simulink model "UR5_CB3_admittance_template"  (R2020b)
settings: Solver=FixedStepAuto  StartTime=0.0  StopTime=30  FixedStep=1/500  MaxStep=1e-2  RelTol=1e-3
model workspace: external: MATLAB File UR5_CB3Params.m (data not in the file)
values from neighbouring files (symbols this model uses):
  a = [0 -0.425 -0.39225 0 0 0]    [UR5_CB3Params.m]
  alpha = [1.5707963267948966 0 0 1.5707963267948966 -1.5707963267948966           0]    [UR5_CB3Params.m]
  d = [0.089159 0 0 0.10915 0.09465 0.0823]    [UR5_CB3Params.m]
  m1 = 3.7    [UR5_CB3Params.m]
  m2 = 8.393    [UR5_CB3Params.m]
  m3 = 2.33    [UR5_CB3Params.m]
  m4 = 1.219    [UR5_CB3Params.m]
  m5 = 1.219    [UR5_CB3Params.m]
  m6 = 0.1879    [UR5_CB3Params.m]
  q0 = [1;1;1;1;1;1]    [UR5_CB3Params.m]
  UR5_CB3Data = struct    [UR5_CB3Params.m]
undefined symbols (not defined in the file or in its folder): Do, Kd, Ko, Kp, Md, Mo, X, Y, Z
libraries: sm_lib x154, nesl_utility x19
(part 3 of 3)

== system UR5_CB3_admittance_template/UR5 (CB3)/Link 3/Link 3/x31101_Support_14_RIGID ==
  ReferenceFrame : sm_lib/Frames and Transforms/Reference Frame
  Solid : sm_lib/Body Elements/File Solid  ExtGeomFileName=31101_Support_ipt_da604d82.STEP  UnitType=FromFile  ExtGeomFileUnits=m  StepReaderType=HEX  ExportConvexHullGeometry=off  InertiaType=Custom  Mass=UR5_CB3Data.Solid(8).mass  MassUnits=lbm  CenterOfMass=UR5_CB3Data.Solid(8).CoM  CenterOfMassUnits=mm  MomentsOfInertia=UR5_CB3Data.Solid(8).MoI  MomentsOfInertiaUnits=lbm*mm^2  ProductsOfInertia=UR5_CB3Data.Solid(8).PoI  ProductsOfInertiaUnits=lbm*mm^2  BasedOnType=Density  Density=1000  DensityUnits=kg/m^3  DoExposeReferenceFrame=on  SerializedFrames=<Frames/>  GraphicType=FromGeometry  MarkerShape=Sphere  MarkerSize=10  GraphicVisPropType=SimpleVisualProperties  GraphicDiffuseColor=UR5_CB3Data.Solid(8).color  GraphicSpecularColor=[0.5 0.5 0.5 1.0]  GraphicAmbientColor=[0.15 0.15 0.15 1.0]  GraphicEmissiveColor=[0.0 0.0 0.0 1.0]  GraphicShininess=75  GraphicOpacity=UR5_CB3Data.Solid(8).opacity
  F : PMIOPort  Side=Left
  connections:
  Solid/RConn1 -- ReferenceFrame/RConn1 -- F/RConn1

== system UR5_CB3_admittance_template/UR5 (CB3)/Link 3/Link 3/x31105_Support_24_RIGID ==
  ReferenceFrame : sm_lib/Frames and Transforms/Reference Frame
  Solid : sm_lib/Body Elements/File Solid  ExtGeomFileName=31105_Support_ipt_79716e66.STEP  UnitType=FromFile  ExtGeomFileUnits=m  StepReaderType=HEX  ExportConvexHullGeometry=off  InertiaType=Custom  Mass=UR5_CB3Data.Solid(12).mass  MassUnits=lbm  CenterOfMass=UR5_CB3Data.Solid(12).CoM  CenterOfMassUnits=mm  MomentsOfInertia=UR5_CB3Data.Solid(12).MoI  MomentsOfInertiaUnits=lbm*mm^2  ProductsOfInertia=UR5_CB3Data.Solid(12).PoI  ProductsOfInertiaUnits=lbm*mm^2  BasedOnType=Density  Density=1000  DensityUnits=kg/m^3  DoExposeReferenceFrame=on  SerializedFrames=<Frames/>  GraphicType=FromGeometry  MarkerShape=Sphere  MarkerSize=10  GraphicVisPropType=SimpleVisualProperties  GraphicDiffuseColor=UR5_CB3Data.Solid(12).color  GraphicSpecularColor=[0.5 0.5 0.5 1.0]  GraphicAmbientColor=[0.15 0.15 0.15 1.0]  GraphicEmissiveColor=[0.0 0.0 0.0 1.0]  GraphicShininess=75  GraphicOpacity=UR5_CB3Data.Solid(12).opacity
  F : PMIOPort  Side=Left
  connections:
  Solid/RConn1 -- ReferenceFrame/RConn1 -- F/RConn1

== system UR5_CB3_admittance_template/UR5 (CB3)/Link 3/Link 3/x31106_Support_13_RIGID ==
  ReferenceFrame : sm_lib/Frames and Transforms/Reference Frame
  Solid : sm_lib/Body Elements/File Solid  ExtGeomFileName=31106_Support_ipt_3245b488.STEP  UnitType=FromFile  ExtGeomFileUnits=m  StepReaderType=HEX  ExportConvexHullGeometry=off  InertiaType=Custom  Mass=UR5_CB3Data.Solid(7).mass  MassUnits=lbm  CenterOfMass=UR5_CB3Data.Solid(7).CoM  CenterOfMassUnits=mm  MomentsOfInertia=UR5_CB3Data.Solid(7).MoI  MomentsOfInertiaUnits=lbm*mm^2  ProductsOfInertia=UR5_CB3Data.Solid(7).PoI  ProductsOfInertiaUnits=lbm*mm^2  BasedOnType=Density  Density=1000  DensityUnits=kg/m^3  DoExposeReferenceFrame=on  SerializedFrames=<Frames/>  GraphicType=FromGeometry  MarkerShape=Sphere  MarkerSize=10  GraphicVisPropType=SimpleVisualProperties  GraphicDiffuseColor=UR5_CB3Data.Solid(7).color  GraphicSpecularColor=[0.5 0.5 0.5 1.0]  GraphicAmbientColor=[0.15 0.15 0.15 1.0]  GraphicEmissiveColor=[0.0 0.0 0.0 1.0]  GraphicShininess=75  GraphicOpacity=UR5_CB3Data.Solid(7).opacity
  F : PMIOPort  Side=Left
  connections:
  Solid/RConn1 -- ReferenceFrame/RConn1 -- F/RConn1

== system UR5_CB3_admittance_template/UR5 (CB3)/Link 3/Link 3/x31362_Support_27_RIGID ==
  ReferenceFrame : sm_lib/Frames and Transforms/Reference Frame
  Solid : sm_lib/Body Elements/File Solid  ExtGeomFileName=31362_Support_ipt_dfed11ef.STEP  UnitType=FromFile  ExtGeomFileUnits=m  StepReaderType=HEX  ExportConvexHullGeometry=off  InertiaType=Custom  Mass=UR5_CB3Data.Solid(14).mass  MassUnits=lbm  CenterOfMass=UR5_CB3Data.Solid(14).CoM  CenterOfMassUnits=mm  MomentsOfInertia=UR5_CB3Data.Solid(14).MoI  MomentsOfInertiaUnits=lbm*mm^2  ProductsOfInertia=UR5_CB3Data.Solid(14).PoI  ProductsOfInertiaUnits=lbm*mm^2  BasedOnType=Density  Density=1000  DensityUnits=kg/m^3  DoExposeReferenceFrame=on  SerializedFrames=<Frames/>  GraphicType=FromGeometry  MarkerShape=Sphere  MarkerSize=10  GraphicVisPropType=SimpleVisualProperties  GraphicDiffuseColor=UR5_CB3Data.Solid(14).color  GraphicSpecularColor=[0.5 0.5 0.5 1.0]  GraphicAmbientColor=[0.15 0.15 0.15 1.0]  GraphicEmissiveColor=[0.0 0.0 0.0 1.0]  GraphicShininess=75  GraphicOpacity=UR5_CB3Data.Solid(14).opacity
  F : PMIOPort  Side=Left
  connections:
  Solid/RConn1 -- ReferenceFrame/RConn1 -- F/RConn1

== system UR5_CB3_admittance_template/UR5 (CB3)/Link 3/Link 3/x33115_Support_32_RIGID ==
  ReferenceFrame : sm_lib/Frames and Transforms/Reference Frame
  Solid : sm_lib/Body Elements/File Solid  ExtGeomFileName=33115_Support_ipt_5ce5d1d.STEP  UnitType=FromFile  ExtGeomFileUnits=m  StepReaderType=HEX  ExportConvexHullGeometry=off  InertiaType=Custom  Mass=UR5_CB3Data.Solid(16).mass  MassUnits=lbm  CenterOfMass=UR5_CB3Data.Solid(16).CoM  CenterOfMassUnits=mm  MomentsOfInertia=UR5_CB3Data.Solid(16).MoI  MomentsOfInertiaUnits=lbm*mm^2  ProductsOfInertia=UR5_CB3Data.Solid(16).PoI  ProductsOfInertiaUnits=lbm*mm^2  BasedOnType=Density  Density=1000  DensityUnits=kg/m^3  DoExposeReferenceFrame=on  SerializedFrames=<Frames/>  GraphicType=FromGeometry  MarkerShape=Sphere  MarkerSize=10  GraphicVisPropType=SimpleVisualProperties  GraphicDiffuseColor=UR5_CB3Data.Solid(16).color  GraphicSpecularColor=[0.5 0.5 0.5 1.0]  GraphicAmbientColor=[0.15 0.15 0.15 1.0]  GraphicEmissiveColor=[0.0 0.0 0.0 1.0]  GraphicShininess=75  GraphicOpacity=UR5_CB3Data.Solid(16).opacity
  F : PMIOPort  Side=Left
  connections:
  Solid/RConn1 -- ReferenceFrame/RConn1 -- F/RConn1

== system UR5_CB3_admittance_template/UR5 (CB3)/Link 3/Link 3/x33116_Support_31_RIGID ==
  ReferenceFrame : sm_lib/Frames and Transforms/Reference Frame
  Solid : sm_lib/Body Elements/File Solid  ExtGeomFileName=33116_Support_ipt_643963fc.STEP  UnitType=FromFile  ExtGeomFileUnits=m  StepReaderType=HEX  ExportConvexHullGeometry=off  InertiaType=Custom  Mass=UR5_CB3Data.Solid(15).mass  MassUnits=lbm  CenterOfMass=UR5_CB3Data.Solid(15).CoM  CenterOfMassUnits=mm  MomentsOfInertia=UR5_CB3Data.Solid(15).MoI  MomentsOfInertiaUnits=lbm*mm^2  ProductsOfInertia=UR5_CB3Data.Solid(15).PoI  ProductsOfInertiaUnits=lbm*mm^2  BasedOnType=Density  Density=1000  DensityUnits=kg/m^3  DoExposeReferenceFrame=on  SerializedFrames=<Frames/>  GraphicType=FromGeometry  MarkerShape=Sphere  MarkerSize=10  GraphicVisPropType=SimpleVisualProperties  GraphicDiffuseColor=UR5_CB3Data.Solid(15).color  GraphicSpecularColor=[0.5 0.5 0.5 1.0]  GraphicAmbientColor=[0.15 0.15 0.15 1.0]  GraphicEmissiveColor=[0.0 0.0 0.0 1.0]  GraphicShininess=75  GraphicOpacity=UR5_CB3Data.Solid(15).opacity
  F : PMIOPort  Side=Left
  connections:
  Solid/RConn1 -- ReferenceFrame/RConn1 -- F/RConn1

== system UR5_CB3_admittance_template/UR5 (CB3)/Link 3/Link 3/x33303_Support_11_RIGID ==
  ReferenceFrame : sm_lib/Frames and Transforms/Reference Frame
  Solid : sm_lib/Body Elements/File Solid  ExtGeomFileName=33303_Support_ipt_9d9e7990.STEP  UnitType=FromFile  ExtGeomFileUnits=m  StepReaderType=HEX  ExportConvexHullGeometry=off  InertiaType=Custom  Mass=UR5_CB3Data.Solid(2).mass  MassUnits=lbm  CenterOfMass=UR5_CB3Data.Solid(2).CoM  CenterOfMassUnits=mm  MomentsOfInertia=UR5_CB3Data.Solid(2).MoI  MomentsOfInertiaUnits=lbm*mm^2  ProductsOfInertia=UR5_CB3Data.Solid(2).PoI  ProductsOfInertiaUnits=lbm*mm^2  BasedOnType=Density  Density=1000  DensityUnits=kg/m^3  DoExposeReferenceFrame=on  SerializedFrames=<Frames/>  GraphicType=FromGeometry  MarkerShape=Sphere  MarkerSize=10  GraphicVisPropType=SimpleVisualProperties  GraphicDiffuseColor=UR5_CB3Data.Solid(2).color  GraphicSpecularColor=[0.5 0.5 0.5 1.0]  GraphicAmbientColor=[0.15 0.15 0.15 1.0]  GraphicEmissiveColor=[0.0 0.0 0.0 1.0]  GraphicShininess=75  GraphicOpacity=UR5_CB3Data.Solid(2).opacity
  F : PMIOPort  Side=Left
  connections:
  Solid/RConn1 -- ReferenceFrame/RConn1 -- F/RConn1

== system UR5_CB3_admittance_template/UR5 (CB3)/Link 3/Link 3/x34111_Support_15_RIGID ==
  ReferenceFrame : sm_lib/Frames and Transforms/Reference Frame
  Solid : sm_lib/Body Elements/File Solid  ExtGeomFileName=34111_Support_ipt_45739413.STEP  UnitType=FromFile  ExtGeomFileUnits=m  StepReaderType=HEX  ExportConvexHullGeometry=off  InertiaType=Custom  Mass=UR5_CB3Data.Solid(9).mass  MassUnits=lbm  CenterOfMass=UR5_CB3Data.Solid(9).CoM  CenterOfMassUnits=mm  MomentsOfInertia=UR5_CB3Data.Solid(9).MoI  MomentsOfInertiaUnits=lbm*mm^2  ProductsOfInertia=UR5_CB3Data.Solid(9).PoI  ProductsOfInertiaUnits=lbm*mm^2  BasedOnType=Density  Density=1000  DensityUnits=kg/m^3  DoExposeReferenceFrame=on  SerializedFrames=<Frames/>  GraphicType=FromGeometry  MarkerShape=Sphere  MarkerSize=10  GraphicVisPropType=SimpleVisualProperties  GraphicDiffuseColor=UR5_CB3Data.Solid(9).color  GraphicSpecularColor=[0.5 0.5 0.5 1.0]  GraphicAmbientColor=[0.15 0.15 0.15 1.0]  GraphicEmissiveColor=[0.0 0.0 0.0 1.0]  GraphicShininess=75  GraphicOpacity=UR5_CB3Data.Solid(9).opacity
  F : PMIOPort  Side=Left
  connections:
  Solid/RConn1 -- ReferenceFrame/RConn1 -- F/RConn1

== system UR5_CB3_admittance_template/UR5 (CB3)/Link 4/Link 4/x31101_Support_16_RIGID ==
  ReferenceFrame : sm_lib/Frames and Transforms/Reference Frame
  Solid : sm_lib/Body Elements/File Solid  ExtGeomFileName=31101_Support_ipt_da604d82.STEP  UnitType=FromFile  ExtGeomFileUnits=m  StepReaderType=HEX  ExportConvexHullGeometry=off  InertiaType=Custom  Mass=UR5_CB3Data.Solid(8).mass  MassUnits=lbm  CenterOfMass=UR5_CB3Data.Solid(8).CoM  CenterOfMassUnits=mm  MomentsOfInertia=UR5_CB3Data.Solid(8).MoI  MomentsOfInertiaUnits=lbm*mm^2  ProductsOfInertia=UR5_CB3Data.Solid(8).PoI  ProductsOfInertiaUnits=lbm*mm^2  BasedOnType=Density  Density=1000  DensityUnits=kg/m^3  DoExposeReferenceFrame=on  SerializedFrames=<Frames/>  GraphicType=FromGeometry  MarkerShape=Sphere  MarkerSize=10  GraphicVisPropType=SimpleVisualProperties  GraphicDiffuseColor=UR5_CB3Data.Solid(8).color  GraphicSpecularColor=[0.5 0.5 0.5 1.0]  GraphicAmbientColor=[0.15 0.15 0.15 1.0]  GraphicEmissiveColor=[0.0 0.0 0.0 1.0]  GraphicShininess=75  GraphicOpacity=UR5_CB3Data.Solid(8).opacity
  F : PMIOPort  Side=Left
  connections:
  Solid/RConn1 -- ReferenceFrame/RConn1 -- F/RConn1

== system UR5_CB3_admittance_template/UR5 (CB3)/Link 4/Link 4/x31132_Support_25_RIGID ==
  ReferenceFrame : sm_lib/Frames and Transforms/Reference Frame
  Solid : sm_lib/Body Elements/File Solid  ExtGeomFileName=31132_Support_ipt_77457c2f.STEP  UnitType=FromFile  ExtGeomFileUnits=m  StepReaderType=HEX  ExportConvexHullGeometry=off  InertiaType=Custom  Mass=UR5_CB3Data.Solid(13).mass  MassUnits=lbm  CenterOfMass=UR5_CB3Data.Solid(13).CoM  CenterOfMassUnits=mm  MomentsOfInertia=UR5_CB3Data.Solid(13).MoI  MomentsOfInertiaUnits=lbm*mm^2  ProductsOfInertia=UR5_CB3Data.Solid(13).PoI  ProductsOfInertiaUnits=lbm*mm^2  BasedOnType=Density  Density=1000  DensityUnits=kg/m^3  DoExposeReferenceFrame=on  SerializedFrames=<Frames/>  GraphicType=FromGeometry  MarkerShape=Sphere  MarkerSize=10  GraphicVisPropType=SimpleVisualProperties  GraphicDiffuseColor=UR5_CB3Data.Solid(13).color  GraphicSpecularColor=[0.5 0.5 0.5 1.0]  GraphicAmbientColor=[0.15 0.15 0.15 1.0]  GraphicEmissiveColor=[0.0 0.0 0.0 1.0]  GraphicShininess=75  GraphicOpacity=UR5_CB3Data.Solid(13).opacity
  F : PMIOPort  Side=Left
  connections:
  Solid/RConn1 -- ReferenceFrame/RConn1 -- F/RConn1

== system UR5_CB3_admittance_template/UR5 (CB3)/Link 4/Link 4/x33103_Support_20_RIGID ==
  ReferenceFrame : sm_lib/Frames and Transforms/Reference Frame
  Solid : sm_lib/Body Elements/File Solid  ExtGeomFileName=33103_Support_ipt_c3be2011.STEP  UnitType=FromFile  ExtGeomFileUnits=m  StepReaderType=HEX  ExportConvexHullGeometry=off  InertiaType=Custom  Mass=UR5_CB3Data.Solid(10).mass  MassUnits=lbm  CenterOfMass=UR5_CB3Data.Solid(10).CoM  CenterOfMassUnits=mm  MomentsOfInertia=UR5_CB3Data.Solid(10).MoI  MomentsOfInertiaUnits=lbm*mm^2  ProductsOfInertia=UR5_CB3Data.Solid(10).PoI  ProductsOfInertiaUnits=lbm*mm^2  BasedOnType=Density  Density=1000  DensityUnits=kg/m^3  DoExposeReferenceFrame=on  SerializedFrames=<Frames/>  GraphicType=FromGeometry  MarkerShape=Sphere  MarkerSize=10  GraphicVisPropType=SimpleVisualProperties  GraphicDiffuseColor=UR5_CB3Data.Solid(10).color  GraphicSpecularColor=[0.5 0.5 0.5 1.0]  GraphicAmbientColor=[0.15 0.15 0.15 1.0]  GraphicEmissiveColor=[0.0 0.0 0.0 1.0]  GraphicShininess=75  GraphicOpacity=UR5_CB3Data.Solid(10).opacity
  F : PMIOPort  Side=Left
  connections:
  Solid/RConn1 -- ReferenceFrame/RConn1 -- F/RConn1

== system UR5_CB3_admittance_template/UR5 (CB3)/Link 4/Link 4/x33116_Support_30_RIGID ==
  ReferenceFrame : sm_lib/Frames and Transforms/Reference Frame
  Solid : sm_lib/Body Elements/File Solid  ExtGeomFileName=33116_Support_ipt_643963fc.STEP  UnitType=FromFile  ExtGeomFileUnits=m  StepReaderType=HEX  ExportConvexHullGeometry=off  InertiaType=Custom  Mass=UR5_CB3Data.Solid(15).mass  MassUnits=lbm  CenterOfMass=UR5_CB3Data.Solid(15).CoM  CenterOfMassUnits=mm  MomentsOfInertia=UR5_CB3Data.Solid(15).MoI  MomentsOfInertiaUnits=lbm*mm^2  ProductsOfInertia=UR5_CB3Data.Solid(15).PoI  ProductsOfInertiaUnits=lbm*mm^2  BasedOnType=Density  Density=1000  DensityUnits=kg/m^3  DoExposeReferenceFrame=on  SerializedFrames=<Frames/>  GraphicType=FromGeometry  MarkerShape=Sphere  MarkerSize=10  GraphicVisPropType=SimpleVisualProperties  GraphicDiffuseColor=UR5_CB3Data.Solid(15).color  GraphicSpecularColor=[0.5 0.5 0.5 1.0]  GraphicAmbientColor=[0.15 0.15 0.15 1.0]  GraphicEmissiveColor=[0.0 0.0 0.0 1.0]  GraphicShininess=75  GraphicOpacity=UR5_CB3Data.Solid(15).opacity
  F : PMIOPort  Side=Left
  connections:
  Solid/RConn1 -- ReferenceFrame/RConn1 -- F/RConn1

== system UR5_CB3_admittance_template/UR5 (CB3)/Link 4/Link 4/x34111_Support_17_RIGID ==
  ReferenceFrame : sm_lib/Frames and Transforms/Reference Frame
  Solid : sm_lib/Body Elements/File Solid  ExtGeomFileName=34111_Support_ipt_45739413.STEP  UnitType=FromFile  ExtGeomFileUnits=m  StepReaderType=HEX  ExportConvexHullGeometry=off  InertiaType=Custom  Mass=UR5_CB3Data.Solid(9).mass  MassUnits=lbm  CenterOfMass=UR5_CB3Data.Solid(9).CoM  CenterOfMassUnits=mm  MomentsOfInertia=UR5_CB3Data.Solid(9).MoI  MomentsOfInertiaUnits=lbm*mm^2  ProductsOfInertia=UR5_CB3Data.Solid(9).PoI  ProductsOfInertiaUnits=lbm*mm^2  BasedOnType=Density  Density=1000  DensityUnits=kg/m^3  DoExposeReferenceFrame=on  SerializedFrames=<Frames/>  GraphicType=FromGeometry  MarkerShape=Sphere  MarkerSize=10  GraphicVisPropType=SimpleVisualProperties  GraphicDiffuseColor=UR5_CB3Data.Solid(9).color  GraphicSpecularColor=[0.5 0.5 0.5 1.0]  GraphicAmbientColor=[0.15 0.15 0.15 1.0]  GraphicEmissiveColor=[0.0 0.0 0.0 1.0]  GraphicShininess=75  GraphicOpacity=UR5_CB3Data.Solid(9).opacity
  F : PMIOPort  Side=Left
  connections:
  Solid/RConn1 -- ReferenceFrame/RConn1 -- F/RConn1

== system UR5_CB3_admittance_template/UR5 (CB3)/Link 5/Link 5/x31101_Support_18_RIGID ==
  ReferenceFrame : sm_lib/Frames and Transforms/Reference Frame
  Solid : sm_lib/Body Elements/File Solid  ExtGeomFileName=31101_Support_ipt_da604d82.STEP  UnitType=FromFile  ExtGeomFileUnits=m  StepReaderType=HEX  ExportConvexHullGeometry=off  InertiaType=Custom  Mass=UR5_CB3Data.Solid(8).mass  MassUnits=lbm  CenterOfMass=UR5_CB3Data.Solid(8).CoM  CenterOfMassUnits=mm  MomentsOfInertia=UR5_CB3Data.Solid(8).MoI  MomentsOfInertiaUnits=lbm*mm^2  ProductsOfInertia=UR5_CB3Data.Solid(8).PoI  ProductsOfInertiaUnits=lbm*mm^2  BasedOnType=Density  Density=1000  DensityUnits=kg/m^3  DoExposeReferenceFrame=on  SerializedFrames=<Frames/>  GraphicType=FromGeometry  MarkerShape=Sphere  MarkerSize=10  GraphicVisPropType=SimpleVisualProperties  GraphicDiffuseColor=UR5_CB3Data.Solid(8).color  GraphicSpecularColor=[0.5 0.5 0.5 1.0]  GraphicAmbientColor=[0.15 0.15 0.15 1.0]  GraphicEmissiveColor=[0.0 0.0 0.0 1.0]  GraphicShininess=75  GraphicOpacity=UR5_CB3Data.Solid(8).opacity
  F : PMIOPort  Side=Left
  connections:
  Solid/RConn1 -- ReferenceFrame/RConn1 -- F/RConn1

== system UR5_CB3_admittance_template/UR5 (CB3)/Link 5/Link 5/x31132_Support_26_RIGID ==
  ReferenceFrame : sm_lib/Frames and Transforms/Reference Frame
  Solid : sm_lib/Body Elements/File Solid  ExtGeomFileName=31132_Support_ipt_77457c2f.STEP  UnitType=FromFile  ExtGeomFileUnits=m  StepReaderType=HEX  ExportConvexHullGeometry=off  InertiaType=Custom  Mass=UR5_CB3Data.Solid(13).mass  MassUnits=lbm  CenterOfMass=UR5_CB3Data.Solid(13).CoM  CenterOfMassUnits=mm  MomentsOfInertia=UR5_CB3Data.Solid(13).MoI  MomentsOfInertiaUnits=lbm*mm^2  ProductsOfInertia=UR5_CB3Data.Solid(13).PoI  ProductsOfInertiaUnits=lbm*mm^2  BasedOnType=Density  Density=1000  DensityUnits=kg/m^3  DoExposeReferenceFrame=on  SerializedFrames=<Frames/>  GraphicType=FromGeometry  MarkerShape=Sphere  MarkerSize=10  GraphicVisPropType=SimpleVisualProperties  GraphicDiffuseColor=UR5_CB3Data.Solid(13).color  GraphicSpecularColor=[0.5 0.5 0.5 1.0]  GraphicAmbientColor=[0.15 0.15 0.15 1.0]  GraphicEmissiveColor=[0.0 0.0 0.0 1.0]  GraphicShininess=75  GraphicOpacity=UR5_CB3Data.Solid(13).opacity
  F : PMIOPort  Side=Left
  connections:
  Solid/RConn1 -- ReferenceFrame/RConn1 -- F/RConn1

== system UR5_CB3_admittance_template/UR5 (CB3)/Link 5/Link 5/x33103_Support_21_RIGID ==
  ReferenceFrame : sm_lib/Frames and Transforms/Reference Frame
  Solid : sm_lib/Body Elements/File Solid  ExtGeomFileName=33103_Support_ipt_c3be2011.STEP  UnitType=FromFile  ExtGeomFileUnits=m  StepReaderType=HEX  ExportConvexHullGeometry=off  InertiaType=Custom  Mass=UR5_CB3Data.Solid(10).mass  MassUnits=lbm  CenterOfMass=UR5_CB3Data.Solid(10).CoM  CenterOfMassUnits=mm  MomentsOfInertia=UR5_CB3Data.Solid(10).MoI  MomentsOfInertiaUnits=lbm*mm^2  ProductsOfInertia=UR5_CB3Data.Solid(10).PoI  ProductsOfInertiaUnits=lbm*mm^2  BasedOnType=Density  Density=1000  DensityUnits=kg/m^3  DoExposeReferenceFrame=on  SerializedFrames=<Frames/>  GraphicType=FromGeometry  MarkerShape=Sphere  MarkerSize=10  GraphicVisPropType=SimpleVisualProperties  GraphicDiffuseColor=UR5_CB3Data.Solid(10).color  GraphicSpecularColor=[0.5 0.5 0.5 1.0]  GraphicAmbientColor=[0.15 0.15 0.15 1.0]  GraphicEmissiveColor=[0.0 0.0 0.0 1.0]  GraphicShininess=75  GraphicOpacity=UR5_CB3Data.Solid(10).opacity
  F : PMIOPort  Side=Left
  connections:
  Solid/RConn1 -- ReferenceFrame/RConn1 -- F/RConn1

== system UR5_CB3_admittance_template/UR5 (CB3)/Link 5/Link 5/x33116_Support_29_RIGID ==
  ReferenceFrame : sm_lib/Frames and Transforms/Reference Frame
  Solid : sm_lib/Body Elements/File Solid  ExtGeomFileName=33116_Support_ipt_643963fc.STEP  UnitType=FromFile  ExtGeomFileUnits=m  StepReaderType=HEX  ExportConvexHullGeometry=off  InertiaType=Custom  Mass=UR5_CB3Data.Solid(15).mass  MassUnits=lbm  CenterOfMass=UR5_CB3Data.Solid(15).CoM  CenterOfMassUnits=mm  MomentsOfInertia=UR5_CB3Data.Solid(15).MoI  MomentsOfInertiaUnits=lbm*mm^2  ProductsOfInertia=UR5_CB3Data.Solid(15).PoI  ProductsOfInertiaUnits=lbm*mm^2  BasedOnType=Density  Density=1000  DensityUnits=kg/m^3  DoExposeReferenceFrame=on  SerializedFrames=<Frames/>  GraphicType=FromGeometry  MarkerShape=Sphere  MarkerSize=10  GraphicVisPropType=SimpleVisualProperties  GraphicDiffuseColor=UR5_CB3Data.Solid(15).color  GraphicSpecularColor=[0.5 0.5 0.5 1.0]  GraphicAmbientColor=[0.15 0.15 0.15 1.0]  GraphicEmissiveColor=[0.0 0.0 0.0 1.0]  GraphicShininess=75  GraphicOpacity=UR5_CB3Data.Solid(15).opacity
  F : PMIOPort  Side=Left
  connections:
  Solid/RConn1 -- ReferenceFrame/RConn1 -- F/RConn1

== system UR5_CB3_admittance_template/UR5 (CB3)/Link 5/Link 5/x34111_Support_19_RIGID ==
  ReferenceFrame : sm_lib/Frames and Transforms/Reference Frame
  Solid : sm_lib/Body Elements/File Solid  ExtGeomFileName=34111_Support_ipt_45739413.STEP  UnitType=FromFile  ExtGeomFileUnits=m  StepReaderType=HEX  ExportConvexHullGeometry=off  InertiaType=Custom  Mass=UR5_CB3Data.Solid(9).mass  MassUnits=lbm  CenterOfMass=UR5_CB3Data.Solid(9).CoM  CenterOfMassUnits=mm  MomentsOfInertia=UR5_CB3Data.Solid(9).MoI  MomentsOfInertiaUnits=lbm*mm^2  ProductsOfInertia=UR5_CB3Data.Solid(9).PoI  ProductsOfInertiaUnits=lbm*mm^2  BasedOnType=Density  Density=1000  DensityUnits=kg/m^3  DoExposeReferenceFrame=on  SerializedFrames=<Frames/>  GraphicType=FromGeometry  MarkerShape=Sphere  MarkerSize=10  GraphicVisPropType=SimpleVisualProperties  GraphicDiffuseColor=UR5_CB3Data.Solid(9).color  GraphicSpecularColor=[0.5 0.5 0.5 1.0]  GraphicAmbientColor=[0.15 0.15 0.15 1.0]  GraphicEmissiveColor=[0.0 0.0 0.0 1.0]  GraphicShininess=75  GraphicOpacity=UR5_CB3Data.Solid(9).opacity
  F : PMIOPort  Side=Left
  connections:
  Solid/RConn1 -- ReferenceFrame/RConn1 -- F/RConn1

== system UR5_CB3_admittance_template/UR5 (CB3)/Link 6/Link 7/x31008_Support_23_RIGID ==
  ReferenceFrame : sm_lib/Frames and Transforms/Reference Frame
  Solid : sm_lib/Body Elements/File Solid  ExtGeomFileName=31008_Support_ipt_ce5c2366.STEP  UnitType=FromFile  ExtGeomFileUnits=m  StepReaderType=HEX  ExportConvexHullGeometry=off  InertiaType=Custom  Mass=UR5_CB3Data.Solid(11).mass  MassUnits=lbm  CenterOfMass=UR5_CB3Data.Solid(11).CoM  CenterOfMassUnits=mm  MomentsOfInertia=UR5_CB3Data.Solid(11).MoI  MomentsOfInertiaUnits=lbm*mm^2  ProductsOfInertia=UR5_CB3Data.Solid(11).PoI  ProductsOfInertiaUnits=lbm*mm^2  BasedOnType=Density  Density=1000  DensityUnits=kg/m^3  DoExposeReferenceFrame=on  SerializedFrames=<Frames/>  GraphicType=FromGeometry  MarkerShape=Sphere  MarkerSize=10  GraphicVisPropType=SimpleVisualProperties  GraphicDiffuseColor=UR5_CB3Data.Solid(11).color  GraphicSpecularColor=[0.5 0.5 0.5 1.0]  GraphicAmbientColor=[0.15 0.15 0.15 1.0]  GraphicEmissiveColor=[0.0 0.0 0.0 1.0]  GraphicShininess=75  GraphicOpacity=UR5_CB3Data.Solid(11).opacity
  F : PMIOPort  Side=Left
  connections:
  ReferenceFrame/RConn1 -- Solid/RConn1 -- F/RConn1

== system UR5_CB3_admittance_template/UR5 (CB3)/Link 6/Link 7/x33103_Support_22_RIGID ==
  ReferenceFrame : sm_lib/Frames and Transforms/Reference Frame
  Solid : sm_lib/Body Elements/File Solid  ExtGeomFileName=33103_Support_ipt_c3be2011.STEP  UnitType=FromFile  ExtGeomFileUnits=m  StepReaderType=HEX  ExportConvexHullGeometry=off  InertiaType=Custom  Mass=UR5_CB3Data.Solid(10).mass  MassUnits=lbm  CenterOfMass=UR5_CB3Data.Solid(10).CoM  CenterOfMassUnits=mm  MomentsOfInertia=UR5_CB3Data.Solid(10).MoI  MomentsOfInertiaUnits=lbm*mm^2  ProductsOfInertia=UR5_CB3Data.Solid(10).PoI  ProductsOfInertiaUnits=lbm*mm^2  BasedOnType=Density  Density=1000  DensityUnits=kg/m^3  DoExposeReferenceFrame=on  SerializedFrames=<Frames/>  GraphicType=FromGeometry  MarkerShape=Sphere  MarkerSize=10  GraphicVisPropType=SimpleVisualProperties  GraphicDiffuseColor=UR5_CB3Data.Solid(10).color  GraphicSpecularColor=[0.5 0.5 0.5 1.0]  GraphicAmbientColor=[0.15 0.15 0.15 1.0]  GraphicEmissiveColor=[0.0 0.0 0.0 1.0]  GraphicShininess=75  GraphicOpacity=UR5_CB3Data.Solid(10).opacity
  F : PMIOPort  Side=Left
  connections:
  ReferenceFrame/RConn1 -- Solid/RConn1 -- F/RConn1

== matlab function UR5_CB3_admittance_template/Admittance Controller/quat_integrator/quaternion_int ==
  settings: updateMethod=DISCRETE
  data: wcd input; q output
function q = fcn(wcd)

persistent eta eps_cd


if isempty(eta)
    eta = 0;
end

if isempty(eps_cd)
    eps_cd = [1; 0; 0];
end

dt = 1/500;

qt = [eta; eps_cd];

A = [0 -wcd(1) -wcd(2) -wcd(3);
         wcd(1) 0 wcd(3) -wcd(2);
         wcd(2) -wcd(3) 0 wcd(1);
         wcd(3) wcd(2) -wcd(1) 0];
q = (qt + A*qt.*dt)';
q = q/norm(q);
eta = q(1);
eps_cd = q(2:4)';

% wcd = wcd*dt/2;
% R = wcd(1)/2;
% P = wcd(2)/2;
% Y = wcd(3)/2;
% 
% r = [cos(R)*cos(P)*cos(Y)+sin(R)*sin(P)*sin(Y);
%      sin(R)*cos(P)*cos(Y)-cos(R)*sin(P)*sin(Y);
%      cos(R)*sin(P)*cos(Y)+sin(R)*cos(P)*sin(Y);
%      cos(R)*cos(P)*sin(Y)-sin(R)*sin(P)*cos(Y)]';
%  
%  if sum(r == [1 0 0 0]) == 4
%     q = [0 0 0 0];
%     eps_cd = q(2:4);
%     eta = q(1);
%  else
%     r = r/norm(r);
% 
%     q1 = cos(norm(r(2:4)));
%     q2 = r(2:4)/norm(r(2:4))*sin(norm(r(2:4)));
% 
%     q = [q1*eta-dot(q2,eps_cd), (q1*eps_cd + eta*q2 + cross(q2,eps_cd))];
% 
%     q = q/norm(q);
%     eps_cd = q(2:4);
%     eta = q(1);
%  end

== matlab function UR5_CB3_admittance_template/Inverse kinematics/MATLAB Function2 ==
  data: x input; theta_column output; R input
function theta_column  = ikin_5_UR5(x, R)
%IKIN_5_UR5 Summary of this function goes here
gd = [R x; 0 0 0 1];

d1 = 0.089159;
d2 = 0;
d3 = 0;
d4 = 0.10915;
d5 = 0.09465;
d6 = 0.0823;
a1 = 0;
a2 = -0.425;
a3 = -0.39225;
a4 = 0;
a5 = 0;
a6 = 0;
alpha1 = pi/2;
alpha2 = 0;
alpha3 = 0;
alpha4 = pi/2;
alpha5 = -pi/2;
alpha6 = 0;
theta = zeros(6, 8);

% theta1
p05 = gd * [0, 0, -d6, 1]'  - [0, 0, 0, 1]';
angle1 = atan2(p05(2), p05(1));
angle2 = real( acos( complex(d4 / sqrt(p05(2)*p05(2) + p05(1)*p05(1)))) );
solution1=pi/2 + angle1 + angle2;
solution2=pi/2 + angle1 - angle2;

    if solution1 < 0
        solution1 = solution1 + 2*pi;
    elseif solution1 > 2*pi
        solution1 = solution1 - 2*pi;
    end
    if solution2 < 0
        solution2 = solution2 + 2*pi;
    elseif solution2 > 2*pi
        solution2 = solution2 - 2*pi;
    end

% Use function range() to keep the angles in right range
theta(1, 1:4) = solution1;
theta(1, 5:8) = solution2;
theta = real(theta);



% theta5
for i=1:4:5
    T01=trans(1,theta(1,i));
    T10 = inv(T01);
    T16 = T10 * gd;
    p16z = T16(3,4);
    theta(5, i) = real( acos( complex((p16z-d4)/d6) ));
    theta(5, i+1) = real( acos( complex((p16z-d4)/d6) ));
    theta(5, i+2) = real( -acos( complex((p16z-d4)/d6) ));
    theta(5, i+3) = real( -acos( complex((p16z-d4)/d6) ));
end
theta = real(theta);

% theta6
for i=1:8
    T01 = trans(1, theta(1,i));
    T61 = inv(inv(T01)*gd);
    T61zy = T61(2, 3);
    T61zx = T61(1, 3);
    t5 = theta(5, i);
    theta6 = atan2(-T61zy/sin(t5), T61zx/sin(t5));
    theta(6,i)=theta6;
end
theta = real(theta);

% theta3
for i=1:2:8
    T01 = trans(1, theta(1,i));
    T56 = trans(6, theta(6,i));
    T45 = trans(5, theta(5,i));
    T16 = (inv(T01))*gd;
    T14 = T16*(inv(T45*T56));
    p13 = T14 * [0, -d4, 0, 1]' - [0,0,0,1]';
    
    t3p = real( acos(complex( ((norm(p13).^2)-a2*a2-a3*a3)/(2*a2*a3) )) );
    theta(3, i) = t3p;
    theta(3, i+1) = -t3p;
end
theta = real(theta);

% theta2 and theta4
for i=1:8
    % theta2
    T01 = trans(1, theta(1,i));
    T56 = trans(6, theta(6,i));
    T45 = trans(5, theta(5,i));
    T16 = (inv(T01))*gd;
    T14 = T16*(inv(T45*T56));
    p13 = T14 * [0, -d4, 0, 1]' - [0,0,0,1]';
    
    theta(2, i) = -atan2(p13(2), -p13(1))+asin(a3*sin(theta(3,i))/norm(p13));
    % theta4
    T23 = trans(3, theta(3,i));
    T12 = trans(2, theta(2,i));
    T34 = (inv(T12*T23))*T14;
    theta(4, i) = atan2(T34(2,1), T34(1,1));
    
end
theta = real(theta);
theta_column = theta(:,1);
%choose one column of thetas
end


function[G]=trans(i, theta)
% i is the larger frame number
    d1 = 0.089159;
    d2 = 0;
    d3 = 0;
    d4 = 0.10915;
    d5 = 0.09465;
    d6 = 0.0823;
    d=[d1 d2 d3 d4 d5 d6];
    a1 = 0;
    a2 = -0.425;
    a3 = -0.39225;
    a4 = 0;
    a5 = 0;
    a6 = 0;
    a=[a1 a2 a3 a4 a5 a6];
    
    alpha1 = pi/2;
    alpha2 = 0;
    alpha3 = 0;
    alpha4 = pi/2;
    alpha5 = -pi/2;
    alpha6 = 0;
    alpha=[alpha1 alpha2 alpha3 alpha4 alpha5 alpha6];
    
R=ROTX(alpha(i));
g0=eye(4);
g0(1:3,1:3)=R;
g0(1:3,4)=[a(i) 0 d(i)]';
G=twist([0;0;1],[0;0;0],theta)*g0;
end

function matrix = ROTX(r)


matrix = zeros(3,3);

matrix(1,1) = 1;
matrix(1,2) = 0; 
matrix(1,3) = 0;
matrix(2,1) = 0; 
matrix(2,2) = cos(r); 
matrix(2,3) = -sin(r);
matrix(3,1) = 0;
matrix(3,2) = sin(r);
matrix(3,3) = cos(r);
end


function [ G ] = twist( w, q, theta )

    G = eye(4);
    w_hat = zeros(3,3);
    w_hat(1,2) = -w(3);
    w_hat(2,1) = w(3);
    w_hat(1,3) = w(2);
    w_hat(3,1) = -w(2);
    w_hat(2,3) = -w(1);
    w_hat(3,2) = w(1);
    v = -w_hat * q;
    G(1:3, 1:3) = eye(3) + w_hat * sin(theta) + (1-cos(theta)) * w_hat * w_hat;
    G(1:3, 4) = (eye(3)*theta + (1-cos(theta))*w_hat + (theta-sin(theta))*w_hat*w_hat) * v;
end

== matlab function UR5_CB3_admittance_template/Admittance Controller/eps2rpy ==
  data: eps_cd input size=[1 3]; rpy output; eta input
function rpy = fcn(eps_cd, eta)

v = eta;
r = eps_cd;
% S_r = [0 -r(3) r(2);
%        r(3) 0 -r(1);
%        -r(2) r(1) 0]; 

% rot = inv(r*r'+( eye(3)-r*r'*cos(v)+S_r*sin(v) ));
q = [v, r];
if sum(q == [0, 0, 0, 0]) == 4
    rpy = [0, 0, 0];
else
    rpy = quat2eul(q,'XYZ');
end
% rpy = rotm2eul(rot,'XYZ');

== matlab function UR5_CB3_admittance_template/Admittance Controller/Ko_prime ==
  data: eta input; eps_cd input size=[1 3]; Ko_prime output; Ko input
function Ko_prime = fcn(eta, eps_cd,Ko)

if isempty(eps_cd)
    eps_cd = [0 0 0];
end

S_eps = [0 -eps_cd(3) eps_cd(2);
       eps_cd(3) 0 -eps_cd(1);
       -eps_cd(2) eps_cd(1) 0]; 

E = eta*eye(3) - S_eps;

Ko_prime = 2*E*Ko;
